simulink model "OutputToStimAndVisualization"  (R2016b)
settings: Solver=FixedStepDiscrete  StartTime=0.0  StopTime=inf  FixedStep=sCoreParams.core.stepPeriod  RelTol=1e-3  EnableMultiTasking=on
undefined symbols (not defined in the file): sCoreParams
libraries: dspswit3 x5, slrtlib x2
settings Model: DataTypeOverride=Double  MinMaxOverflowLogging=ForceOff  Creator=rzelmann  LastModifiedBy=rzelmann
settings SolverCC: EnableConcurrentExecution=on  ConcurrentTasks=on  AutoInsertRateTranBlk=on
settings DataIOCC: SaveFormat=StructureWithTime  SaveOutput=off  SignalLogging=off  DSMLogging=off  SaveTime=off
settings OptimizationCC: BlockReduction=off  DefaultParameterBehavior=Inlined  LifeSpan=inf
settings DebuggingCC: AllowSymbolicDim=off  SFUnexpectedBacktrackingDiag=warning  SFNoUnconditionalDefaultTransitionDiag=warning  SFExecutionAtInitializationDiag=none
settings HardwareCC: ProdBitPerPointer=32  ProdBitPerSizeT=32  ProdBitPerPtrDiffT=32  ProdLargestAtomicFloat=None  ProdWordSize=32  ProdLongLongMode=on  ProdHWDeviceType=Generic->32-bit x86 compatible
settings ModelReferenceCC: UpdateModelReferenceTargets=Force  ParallelModelReferenceMATLABWorkerInit=Load Top Model  ModelReferenceNumInstancesAllowed=Single  ModelReferencePassRootInputsByReference=off
settings RTWCC: SystemTargetFile=slrt.tlc  TemplateMakefile=slrt_default_tmf  Description=Simulink Real-Time  RTWCompilerOptimization=on
settings CodeAppCC: MaxIdLength=63
settings ConfigComp: CovMetricSettings=dw  CovHtmlReporting=on  CovSaveCumulativeToWorkspaceVar=on  CovSaveSingleToWorkspaceVar=on  CovExternalEMLEnable=off

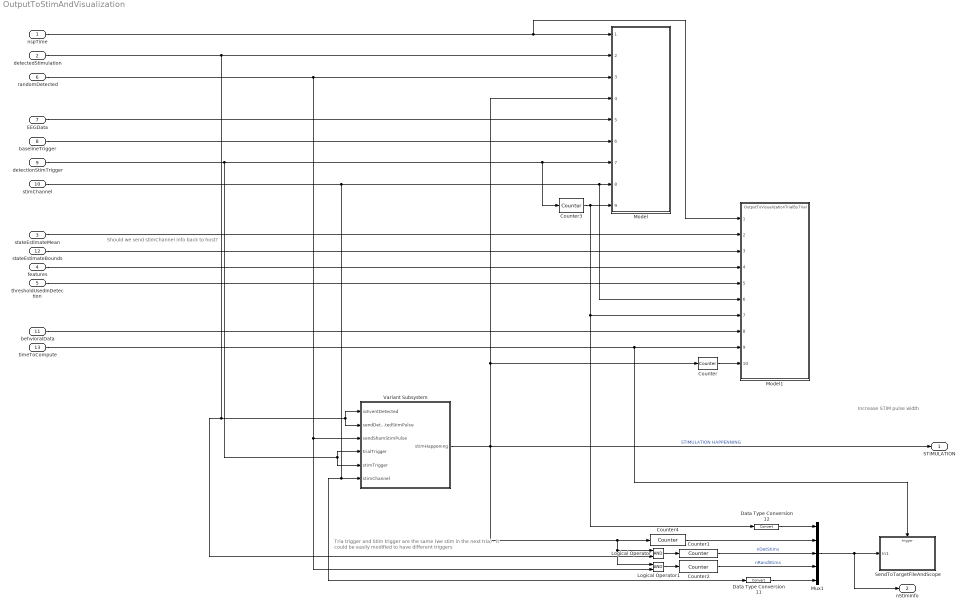
== system OutputToStimAndVisualization ==
  note: Increase STIM pulse width
  note: Should we send stimChannel info back to host?
  note: Tria trigger and Stim trigger are the same (we stim in the next tria)
      | - it could be easily modified to have different triggers
  nspTime : Inport  SampleTime=sCoreParams.core.stepPeriod
  detectedStimulation : Inport  Port=2  SampleTime=sCoreParams.core.stepPeriod
  stateEstimateMean : Inport  Port=3  SampleTime=sCoreParams.core.stepPeriod
  features : Inport  Port=4  SampleTime=sCoreParams.core.stepPeriod
  thresholdUsedInDetection : Inport  Port=5  SampleTime=sCoreParams.core.stepPeriod
  randomDetected : Inport  Port=6  SampleTime=sCoreParams.core.stepPeriod
  EEGData : Inport  Port=7  SampleTime=sCoreParams.core.stepPeriod
  baselineTrigger : Inport  Port=8  SampleTime=sCoreParams.core.stepPeriod
  detectionStimTrigger : Inport  Port=9  SampleTime=sCoreParams.core.stepPeriod
  stimChannel : Inport  Port=10  SampleTime=sCoreParams.core.stepPeriod
  behvioralData : Inport  Port=11  SampleTime=sCoreParams.core.stepPeriod
  stateEstimateBounds : Inport  Port=12  PortDimensions=[1 2]  SampleTime=sCoreParams.core.stepPeriod
  timeToCompute : Inport  Port=13  OutDataTypeStr=boolean  SampleTime=sCoreParams.core.stepPeriod
  Counter{,1..2,4} (4 alike) : dspswit3/Counter  Direction=Up  CountEvent=Rising edge  CounterSize=16 bits  MaxCount=1024  InitialCount=0  Output=Count  HitValue=32  ResetInput=off  SamplesPerFrame=1  Ts=1  CntDtype=double  HitDtype=Logical
  Counter3 : dspswit3/Counter  Direction=Up  CountEvent=Rising edge  CounterSize=User defined  MaxCount=1024  InitialCount=0  Output=Count  HitValue=32  ResetInput=off  SamplesPerFrame=1  Ts=1  CntDtype=double  HitDtype=Logical
  Data Type Conversion11 : DataTypeConversion
  Data Type Conversion12 : DataTypeConversion
  Logical Operator : Logic  IconShape=distinctive  AllPortsSameDT=off  OutDataTypeStr=boolean
  Logical Operator1 : Logic  IconShape=distinctive  AllPortsSameDT=off  OutDataTypeStr=boolean
  Model : ModelReference  ModelNameDialog=OutputToVisualizationContinuous.slx  SimulationMode=Normal  ModelReferenceVersion=1.295
  Model1 : ModelReference  ModelNameDialog=OutputToVisualizationTrialByTrial.slx  SimulationMode=Normal  ModelReferenceVersion=1.288
  Mux1 : Mux  Inputs=5
  SendToTargetFileAndScope : Subsystem
  Variant Subsystem : Subsystem  Variant=on
  STIMULATION : Outport
  nStimInfo : Outport  Port=2
  wires:
  Counter1/1 -> Mux1/3  "nDetStims"
  nspTime/1 -> Model1/1, Model/1
  behvioralData/1 -> Model1/8
  Data Type Conversion11/1 -> Mux1/5
  Variant Subsystem/1(stimHappening) -> STIMULATION/1, Logical Operator1/1, Logical Operator/1, Counter4/1, Counter/1, Model/4  "STIMULATION HAPPENNING"
  Logical Operator1/1 -> Counter2/1
  detectionStimTrigger/1 -> Variant Subsystem/5(stimTrigger), Variant Subsystem/4(trialTrigger), Counter3/1, Model/7
  stimChannel/1 -> Model1/6, Model/8, Data Type Conversion11/1, Variant Subsystem/6(stimChannel)
  baselineTrigger/1 -> Model/6
  Logical Operator/1 -> Counter1/1
  Counter3/1 -> Model/9, Data Type Conversion12/1, Model1/7
  stateEstimateMean/1 -> Model1/2
  thresholdUsedInDetection/1 -> Model1/5
  Mux1/1 -> SendToTargetFileAndScope/1(In1), nStimInfo/1
  EEGData/1 -> Model/5
  Counter2/1 -> Mux1/4  "nRandStims"
  features/1 -> Model1/4
  randomDetected/1 -> Model/3, Logical Operator1/2, Variant Subsystem/3(sendShamStimPulse)
  stateEstimateBounds/1 -> Model1/3
  Counter4/1 -> Mux1/2
  Data Type Conversion12/1 -> Mux1/1
  detectedStimulation/1 -> Model/2, Logical Operator/2, Variant Subsystem/2(sendDetectedStimPulse), Variant Subsystem/1(isEventDetected)
  timeToCompute/1 -> Model1/9, SendToTargetFileAndScope/Trigger
  Counter/1 -> Model1/10

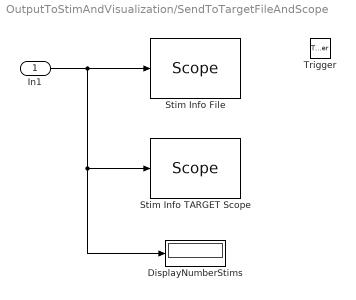
== system OutputToStimAndVisualization/SendToTargetFileAndScope ==
  In1 : Inport
  Trigger : TriggerPort  VariantControl=Variant  PortDimensions=1
  DisplayNumberStims : Display
      settings: Format=decimal (Stored Integer)
  Stim Info File : slrtlib/Displays and Logging/Scope   scopeno=6  scopetype=File  autostart=on  viewmode=Graphical redraw  formatstr='%15.6f'  grid=on  ylimits=[0,0]  nosamples=1000  noprepostsamples=-10  interleave=1  triggermode=FreeRun  triggersignal=1  trigsignalfromport=on  triggerlevel=0.0  triggerslope=Rising  triggerscope=1  triggersample=0  filename=stim_<%%%>.dat  mode=Lazy  writesize=512  autorestart=on  dynamicfilemode=on  maxwritefilesize=512*1024^2
  Stim Info TARGET Scope : slrtlib/Displays and Logging/Scope   scopeno=7  scopetype=Target  autostart=on  viewmode=Numerical  formatstr='%15.0f'  grid=on  ylimits=[0,0]  nosamples=1000  noprepostsamples=0  interleave=1  triggermode=FreeRun  triggersignal=1  trigsignalfromport=on  triggerlevel=0.0  triggerslope=Rising  triggerscope=1  triggersample=0  filename=data.dat  mode=Lazy  writesize=512  autorestart=off  dynamicfilemode=off  maxwritefilesize=512*1024^2
  wires:
  In1/1 -> DisplayNumberStims/1, Stim Info TARGET Scope/1, Stim Info File/1

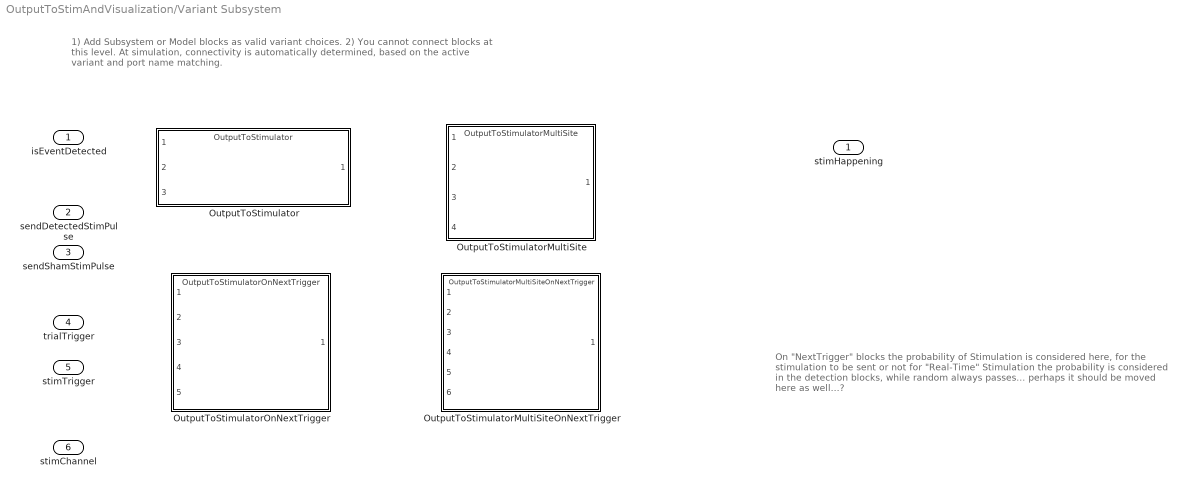
== system OutputToStimAndVisualization/Variant Subsystem ==
  note: On "NextTrigger" blocks the probability of Stimulation is considered here,
      | for the stimulation to be sent or not
      | for "Real-Time" Stimulation the probability is considered in the detection blocks,
      | while random always passes... perhaps it should be moved here as well...?
  note: 1) Add Subsystem or Model blocks as valid variant choices.
      | 2) You cannot connect blocks at this level. At simulation, connectivity is automatically
      | determined, based on the active variant and port name matching.
  isEventDetected : Inport
  sendDetectedStimPulse : Inport  Port=2
  sendShamStimPulse : Inport  Port=3
  trialTrigger : Inport  Port=4
  stimTrigger : Inport  Port=5
  stimChannel : Inport  Port=6  OutDataTypeStr=int32
  OutputToStimulator : ModelReference  ModelNameDialog=OutputToStimulator  SimulationMode=Normal  VariantControl=variantParams_STIMULATION_REALTIME  ModelReferenceVersion=1.34
  OutputToStimulatorMultiSite : ModelReference  ModelNameDialog=OutputToStimulatorMultiSite.slx  SimulationMode=Normal  VariantControl=variantParams_STIMULATION_MULTISITE_REALTIME  ModelReferenceVersion=1.48
  OutputToStimulatorMultiSiteOnNextTrigger : ModelReference  ModelNameDialog=OutputToStimulatorMultiSiteOnNextTrigger.slx  SimulationMode=Normal  VariantControl=variantParams_STIMULATION_MULTISITE_NEXTTRIGGER  ModelReferenceVersion=1.87
  OutputToStimulatorOnNextTrigger : ModelReference  ModelNameDialog=OutputToStimulatorOnNextTrigger  SimulationMode=Normal  VariantControl=variantParams_STIMULATION_ONNEXTTRIGGER  ModelReferenceVersion=1.90
  stimHappening : Outport
